simulink model "MotorXploer"  (R2025a)
settings: Solver=FixedStepAuto  StartTime=0.0  StopTime=inf  FixedStep=0.0005  RelTol=1e-3
undefined symbols (not defined in the file or in its folder): Blocking, LF, Non
libraries: simulink x3, amg_usbconverter_n_connect_lib x3, dspstat3 x1, waijung_addon_module x1
settings Model: Creator=beamk  LastModifiedBy=User

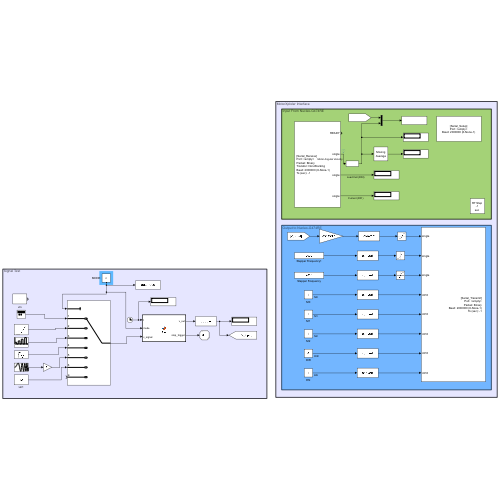
[thumbnail: Simulink's stored preview of the top-level diagram]
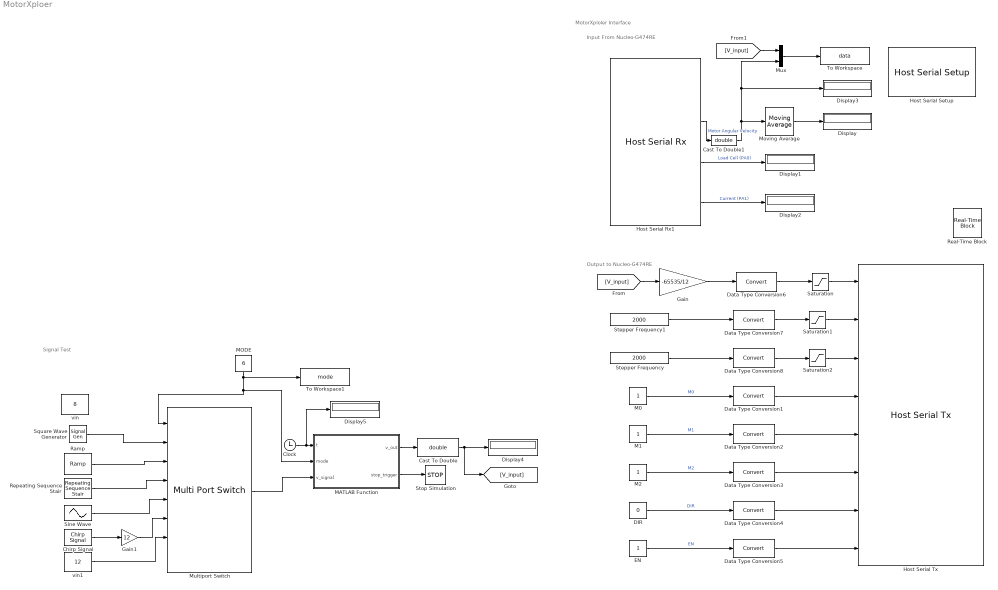
== system MotorXploer ==
  note: Signal Test
  note: Output to Nucleo-G474RE
  note: Input From Nucleo-G474RE
  note: MotorXploler Interface
  Cast To Double : DataTypeConversion  OutDataTypeStr=double  SaturateOnIntegerOverflow=off  RndMeth=Floor
  Cast To Double1 : DataTypeConversion  OutDataTypeStr=double  SaturateOnIntegerOverflow=off  RndMeth=Floor
  Chirp Signal : simulink/Sources/Chirp Signal  f1=0  T=20  f2=pi
  Clock : Clock
      settings: Decimation=5
  DIR : Constant  Value=0
  Data Type Conversion{1..8} (8 alike) : DataTypeConversion  SaturateOnIntegerOverflow=off  RndMeth=Floor
  Display{,1..5} (6 alike) : Display
  EN : Constant
  Gain : Gain  Gain=-65535/12
  Gain1 : Gain  Gain=12
  Host Serial Rx1 : amg_usbconverter_n_connect_lib/Host Serial Rx  conf=rx  port=<auto>  baudrate=2000000  databits=8  parity=None  stopbit=1  flowcontrol=None  transfer=Non-Blocking  timeout=5  packetmode=Binary  enableinitialvalues=off  initialvalues=[]  binheader='25'  binterminator='4E'  porttype_double=0  porttype_single=3  porttype_int8=0  porttype_uint8=0  porttype_int16=0  porttype_uint16=0  porttype_int32=0  porttype_uint32=0  asciiformat='%f,%f,%d,%d'  rx_asciiterminator="LF (0x0A - \"\\n\")"  tx_asciiterminator="CRLF (0x0D 0x0A - \"\\r\\n\")"  sampletime=-1  enablecustomportlabel=off  cinputportlabel=0  coutputportlabel=A  portpinstr=0  blockid=HostSerialRx1  inputporttype=[]  inputportwidth=[]  inputportlabel={}  outputporttype=[3 1 1 1]  outputportwidth=[1 1 1 1]  outputportlabel={'READY','single','single','single'}  compat=0  optionstring=[]  autoport='<empty>'
  Host Serial Setup : amg_usbconverter_n_connect_lib/Host Serial Setup  conf=setup  port=<auto>  baudrate=2000000  databits=8  parity=None  stopbit=1  flowcontrol=None  transfer=Blocking  timeout=2  packetmode=Binary  initialvalues=[]  binheader='7E 7E'  binterminator='03 03'  porttype_double=0  porttype_single=1  porttype_int8=0  porttype_uint8=0  porttype_int16=0  porttype_uint16=0  porttype_int32=0  porttype_uint32=2  asciiformat='%d %u %x'  rx_asciiterminator="CRLF (0x0D 0x0A - \"\\r\\n\")"  tx_asciiterminator="CRLF (0x0D 0x0A - \"\\r\\n\")"  sampletime=-1  enablecustomportlabel=off  cinputportlabel=0  coutputportlabel=A  portpinstr=0  blockid=HostSerialSetup  inputporttype=[]  inputportwidth=[]  inputportlabel={}  outputporttype=[]  outputportwidth=[]  outputportlabel={}  compat=0  optionstring=[]  autoport='<empty>'
  Host Serial Tx : amg_usbconverter_n_connect_lib/Host Serial Tx  conf=tx  port=<auto>  baudrate=2000000  databits=8  parity=None  stopbit=1  flowcontrol=None  transfer=Blocking  timeout=2  packetmode=Binary  initialvalues=[]  binheader='25'  binterminator='4E'  porttype_double=0  porttype_single=3  porttype_int8=0  porttype_uint8=0  porttype_int16=5  porttype_uint16=0  porttype_int32=0  porttype_uint32=0  asciiformat='%d,%f'  rx_asciiterminator="CRLF (0x0D 0x0A - \"\\r\\n\")"  tx_asciiterminator="CRLF (0x0D 0x0A - \"\\r\\n\")"  sampletime=-1  enablecustomportlabel=off  cinputportlabel=0  coutputportlabel=A  portpinstr=0  blockid=HostSerialTx  inputporttype=[1 1 1 4 4 4 4 4]  inputportwidth=[1 1 1 1 1 1 1 1]  inputportlabel={'single','single','single','int16','int16','int16','int16','int16'}  outputporttype=[]  outputportwidth=[]  outputportlabel={}  compat=0  optionstring=[]  autoport='<empty>'
      settings: SourceProductName=aMG USB Converter N
  M0 : Constant
  M1 : Constant
  M2 : Constant
  MATLAB Function : MATLAB Function  TreatAsAtomicUnit=on
  MODE : Constant  Value=6
  Moving Average : dspstat3/Moving Average  Method=Sliding window  ForgettingFactorPort=off  SpecifyWindowLength=on  WindowLength=4  OverlapLength=3  AllowArbitraryInputLength=off  ForgettingFactor=0.9  SimulateUsing=Interpreted execution
  Multiport Switch : MultiPortSwitch  Inputs=6  DataPortForDefault=Additional data port  SaturateOnIntegerOverflow=off  InputSameDT=off
  Mux : Mux  Inputs=2
  Ramp : simulink/Sources/Ramp  slope=3  start=0  InitialOutput=0
  Real-Time Block : waijung_addon_module/Real-Time Block  Priority=0  setting=Default  sampletime=-1
      settings: SourceProductName=Misc
  Repeating Sequence Stair : simulink/Sources/Repeating Sequence Stair  OutValues=[3 0 6 0 9 0 12 0]  tsamp=5  OutMin=[]  OutMax=[]  OutDataTypeStr=double  OutputDataTypeScalingMode=double  OutDataType=fixdt(0,8)  ConRadixGroup=Best Precision: Vector-wise  OutScaling=2^-12
  Saturation : Saturate  UpperLimit=65535  LowerLimit=-65535
  Saturation1 : Saturate  UpperLimit=20000  LowerLimit=0
  Saturation2 : Saturate  UpperLimit=inf  LowerLimit=0
  Sine Wave : Sin  Amplitude=12  Frequency=pi  SampleTime=0
  Square Wave Generator : SignalGenerator  WaveForm=square  Amplitude=6  Frequency=2000
  Stepper Frequency : Constant  Value=2000  OutDataTypeStr=single
  Stepper Frequency1 : Constant  Value=2000  OutDataTypeStr=single
  Stop Simulation : Stop
  To Workspace : ToWorkspace  VariableName=data  SaveFormat=Timeseries  SampleTime=-1
  To Workspace1 : ToWorkspace  VariableName=mode  SaveFormat=Timeseries  SampleTime=-1
  vin : Constant  Value=8
  vin1 : Constant  Value=12
  wires:
  Host Serial Rx1/2 -> Cast To Double1/1  "Motor Angular Velocity"
  Host Serial Rx1/3 -> Display1/1  "Load Cell (PA0)"
  M0/1 -> Data Type Conversion1/1  "M0"
  EN/1 -> Data Type Conversion5/1  "EN"
  DIR/1 -> Data Type Conversion4/1  "DIR"
  M1/1 -> Data Type Conversion2/1  "M1"
  M2/1 -> Data Type Conversion3/1  "M2"
  Stepper Frequency/1 -> Data Type Conversion8/1
  Data Type Conversion1/1 -> Host Serial Tx/4
  Data Type Conversion2/1 -> Host Serial Tx/5
  Data Type Conversion3/1 -> Host Serial Tx/6
  Data Type Conversion4/1 -> Host Serial Tx/7
  Data Type Conversion5/1 -> Host Serial Tx/8
  Data Type Conversion6/1 -> Saturation/1
  Saturation/1 -> Host Serial Tx/1
  Data Type Conversion7/1 -> Saturation1/1
  Data Type Conversion8/1 -> Saturation2/1
  Saturation1/1 -> Host Serial Tx/2
  Saturation2/1 -> Host Serial Tx/3
  Host Serial Rx1/4 -> Display2/1  "Current (PA1)"
  Moving Average/1 -> Display/1
  [V_input] -> Gain/1
  MODE/1 -> Multiport Switch/1, MATLAB Function/2(mode), To Workspace1/1
  Ramp/1 -> Multiport Switch/3
  Repeating Sequence Stair/1 -> Multiport Switch/4
  Sine Wave/1 -> Multiport Switch/5
  Chirp Signal/1 -> Gain1/1
  Gain/1 -> Data Type Conversion6/1
  MATLAB Function/2(stop_trigger) -> Stop Simulation/1
  Multiport Switch/1 -> MATLAB Function/3(v_signal)
  Clock/1 -> Display5/1, MATLAB Function/1(t)
  [V_input] -> Mux/1
  Mux/1 -> To Workspace/1
  MATLAB Function/1(v_out) -> Cast To Double/1
  Cast To Double/1 -> [V_input], Display4/1
  Cast To Double1/1 -> Mux/2, Display3/1, Moving Average/1
  Gain1/1 -> Multiport Switch/6
  vin1/1 -> Multiport Switch/7
  Stepper Frequency1/1 -> Data Type Conversion7/1
  Square Wave Generator/1 -> Multiport Switch/2

== matlab function MotorXploer/MATLAB Function ==
  data: t input; v_out output; mode input; v_signal input; stop_trigger output
function [v_out, stop_trigger] = fcn(t, mode, v_signal)
    % durations = [Step, Ramp, Stair, Sine, Chirp]
    durations = [100, 4, 40, 10, 20,20]; 
    
    % Stage 1: Running
    if t < durations(mode)
        v_out = v_signal;
        stop_trigger = 0;
        
    % Stage 0: Cutoff and Stop
    else
        v_out = 0;           % Forces the motor to stop immediately
        stop_trigger = 1;    % Triggers the Simulink Stop block
    end
end
